simulink model "six_bots_Observer_Collision_MN_VP_NAPF"  (R2021a)
settings: Solver=ode5  StartTime=0.0  StopTime=20  FixedStep=0.005  RelTol=1e-3
(part 4 of 4)

== matlab function six_bots_Observer_Collision_MN_VP_NAPF/Self Calculation 6/Topology changing and APF/Communication based APF ==
  data: x_agents input; F_i output; L_i input
function F_i = commu_based_apf(x_agents, L_i)

%% Notes
% The purpose of this function is perform the APF based on known information

% L_i: a (1,N) vector that represents the communication among agents
% position_agents: the current position of agents

%% Basic parameters
serial_num = 6;
dimension = 3;

alpha = 2;
epsilon_1 = 1.1; % the parameter for the inner boundaries
epsilon_2 = 2; % the parameter for the outer boundaries

%% The info of current agent
Radius=[0.24;0.30;0.23;0.35;0.28;0.25];
r_i = Radius(serial_num);
pos_i = x_agents( (serial_num - 1)*dimension +1 : (serial_num - 1)*dimension +2 );
f_i = [0;0];

for j = 1 : size(L_i,2)
   if j == serial_num   % if it is the agent itself
       f_i = f_i + [0;0];
   else   % if not
       if L_i(j)<0  % if there are connections (meaning it is close enough)
           r_j = Radius(j);    % obtain the radius
           pos_j = x_agents( (j - 1)*dimension +1 : (j - 1)*dimension +2 );
           z_ij = pos_i - pos_j;
           r_in = epsilon_1 * (r_i + r_j);
           r_out = epsilon_2 * (r_i + r_j);
           if norm(z_ij) <= r_out      % if its within the range of APF
               f_ij = alpha* (r_out - norm(z_ij))/(norm(z_ij) - r_in)^2 * z_ij/norm(z_ij);
               f_i = f_i + f_ij;
           end
       end
   end
end

F_i = [f_i;0];
    




end
